simulink model "model_quad_linear_mpc_fail"  (R2021b)
settings: Solver=VariableStepAuto  StartTime=0.0  StopTime=10  RelTol=1e-3
values from neighbouring files (symbols this model uses):
  A = reshape([mt1,mt2,mt3,mt4,mt5,mt6,mt7,mt8],12,12)    [Jacob.m]    (also in Lineared_SS_model.m = reshape([-1.097500e-06;0.000000e+00;0.000000e+00;-4.432200e-; find_optimal_lqr.m = reshape([-1.097500e-06;0.000000e+00;0.000000e+00;-4.432200e-; start_drone.m = zeros(12))
  B = reshape([mt9,mt10],12,4)    [Jacob.m]    (also in Lineared_SS_model.m = reshape([0.000000e+00;0.000000e+00;0.000000e+00;0.000000e+00; find_optimal_lqr.m = reshape([0.000000e+00;0.000000e+00;0.000000e+00;0.000000e+00; nlStateFcn.m = [0 0 0]; start_drone.m = zeros(12,4))
libraries: mpclib x1
settings Model: Creator=Elena  LastModifiedBy=Elena

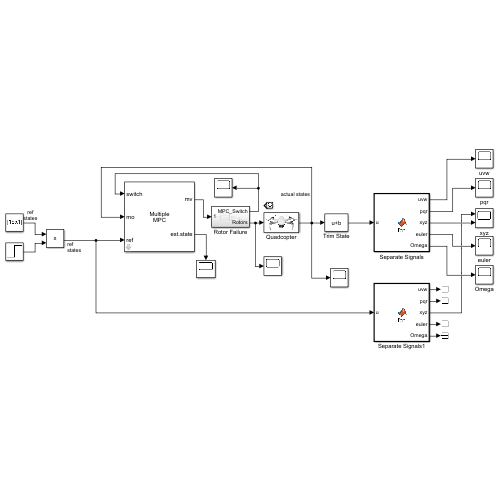
[thumbnail: Simulink's stored preview of the top-level diagram]
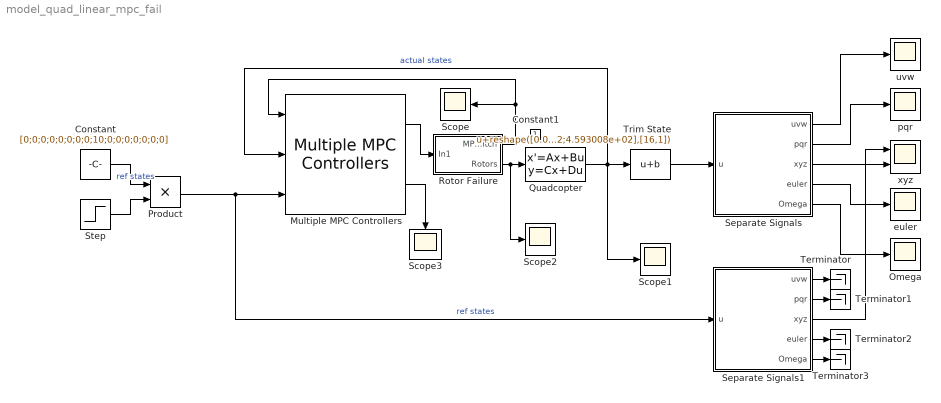
== system model_quad_linear_mpc_fail ==
  Constant : Constant  Value=[0;0;0;0;0;0;0;0;10;0;0;0;0;0;0;0]
  Constant1 : Constant
  Multiple MPC Controllers : mpclib/Multiple MPC Controllers  mpcobjs={'mpc_l','mpc_l_fail_1','mpc_l_fail_2','mpc_l_fail_3','mpc_l_fail_4'}  x0s={'[]','[]','[]','[]','[]'}  Nmpc=1  theMPC=1  nmv=1  nmo=1  nmd=1  nts=1  md_inport_multiple=off  mv_inport_multiple=off  uref_inport_multiple=off  return_cost_multiple=off  return_mvseq_multiple=off  return_qpstatus_multiple=off  return_xseq_multiple=off  return_state_multiple=on  return_ovseq_multiple=off  state_inport_multiple=off  umin_inport_multiple=off  umax_inport_multiple=off  ymin_inport_multiple=off  ymax_inport_multiple=off  ywt_inport_multiple=off  uwt_inport_multiple=off  duwt_inport_multiple=off  rhoeps_inport_multiple=off  BlockDataType_multiple=double  SampleTimeInherited_multiple=off
      settings: SourceProductBaseCode=MP
  Omega : Scope
  Product : Product
  Quadcopter : StateSpace  A=A  B=B  C=eye(16)  D=zeros(16,4)  InitialCondition=0
      mask Display: image('drone_model.png'); % Use "Edit Image" on toolstrip to change.
  Rotor Failure : Subsystem
  Scope{,1..3} (4 alike) : Scope
  Separate Signals : MATLAB Function  TreatAsAtomicUnit=on
  Separate Signals1 : MATLAB Function  TreatAsAtomicUnit=on
  Step : Step  SampleTime=0
  Terminator{,1..3} (4 alike) : Terminator
  Trim State : Bias  Bias=reshape([0.000000e+00;0.000000e+00;0.000000e+00;0.000000e+00;0.000000e+00;0.000000e+00;0.000000e+00;0.000000e+00;0.000000e+00;0.000000e+00;0.000000e+00;0.000000e+00;0;4.593008e+02;4.593008e+02;4.593008e+02],[16,1])
  euler : Scope
  pqr : Scope
  uvw : Scope
  xyz : Scope  NumInputPorts=2
  wires:
  Step/1 -> Product/2
  Quadcopter/1 -> Multiple MPC Controllers/2, Trim State/1, Scope1/1  "actual states"
  Separate Signals/3(xyz) -> xyz/2
  Separate Signals/2(pqr) -> pqr/1
  Separate Signals/1(uvw) -> uvw/1
  Separate Signals/4(euler) -> euler/1
  Separate Signals/5(Omega) -> Omega/1
  Trim State/1 -> Separate Signals/1(u)
  Separate Signals1/3(xyz) -> xyz/1
  Separate Signals1/1(uvw) -> Terminator/1
  Separate Signals1/2(pqr) -> Terminator1/1
  Separate Signals1/4(euler) -> Terminator2/1
  Separate Signals1/5(Omega) -> Terminator3/1
  Multiple MPC Controllers/1 -> Rotor Failure/1(In1)
  Product/1 -> Multiple MPC Controllers/3, Separate Signals1/1(u)  "ref states"
  Constant/1 -> Product/1  "ref states"
  Rotor Failure/2(Rotors) -> Scope2/1, Quadcopter/1
  Rotor Failure/1(MPC_Switch) -> Scope/1, Multiple MPC Controllers/1
  Multiple MPC Controllers/2 -> Scope3/1

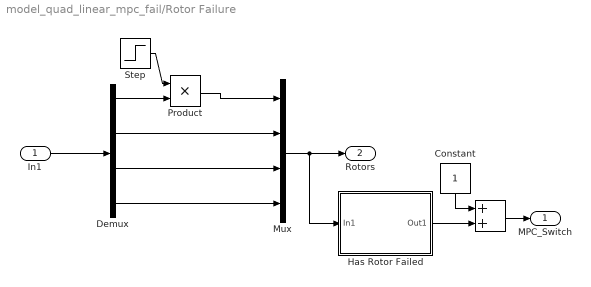
== system model_quad_linear_mpc_fail/Rotor Failure ==
  In1 : Inport
  " " : Sum
  Constant : Constant
  Demux : Demux
  Has Rotor Failed : Subsystem
  Mux : Mux
  Product : Product
  Step : Step  Time=6  Before=1  After=0  SampleTime=0
  MPC_Switch : Outport
  Rotors : Outport  Port=2
  wires:
  In1/1 -> Demux/1
  Demux/3 -> Mux/3
  Demux/4 -> Mux/4
  Product/1 -> Mux/1
  Step/1 -> Product/1
  Demux/2 -> Mux/2
  Demux/1 -> Product/2
  " "/1 -> MPC_Switch/1
  Constant/1 -> " "/1
  Mux/1 -> Has Rotor Failed/1(In1), Rotors/1
  Has Rotor Failed/1(Out1) -> " "/2

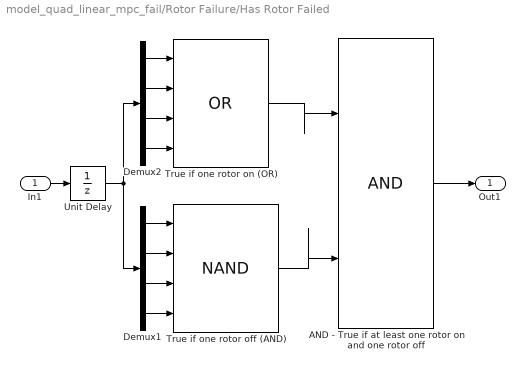
== system model_quad_linear_mpc_fail/Rotor Failure/Has Rotor Failed ==
  In1 : Inport
  "AND - True if at least one rotor on and one rotor off " : Logic  IconShape=distinctive  AllPortsSameDT=off  OutDataTypeStr=boolean
  Demux1 : Demux
  Demux2 : Demux
  True if one rotor off (AND) : Logic  Operator=NAND  Inputs=4  IconShape=distinctive  AllPortsSameDT=off  OutDataTypeStr=boolean
  True if one rotor on (OR) : Logic  Operator=OR  Inputs=4  IconShape=distinctive  AllPortsSameDT=off  OutDataTypeStr=boolean
  Unit Delay : UnitDelay  SampleTime=-1  HasFrameUpgradeWarning=on
  Out1 : Outport
  wires:
  Demux1/2 -> True if one rotor off (AND)/2
  Demux1/4 -> True if one rotor off (AND)/4
  Demux1/1 -> True if one rotor off (AND)/1
  Demux1/3 -> True if one rotor off (AND)/3
  True if one rotor off (AND)/1 -> "AND - True if at least one rotor on and one rotor off "/2
  "AND - True if at least one rotor on and one rotor off "/1 -> Out1/1
  True if one rotor on (OR)/1 -> "AND - True if at least one rotor on and one rotor off "/1
  Unit Delay/1 -> Demux1/1, Demux2/1
  Demux2/3 -> True if one rotor on (OR)/3
  Demux2/1 -> True if one rotor on (OR)/1
  Demux2/4 -> True if one rotor on (OR)/4
  Demux2/2 -> True if one rotor on (OR)/2
  In1/1 -> Unit Delay/1

== matlab function model_quad_linear_mpc_fail/Separate Signals1 ==
  data: u input; uvw output; pqr output; xyz output; euler output; Omega output
function [uvw,pqr,xyz,euler,Omega] = fcn(u)

uvw=u(1:3);
pqr=u((1:3)+3);
xyz=u((1:3)+6);
euler=u((1:3)+9);
Omega=u((1:4)+12);

== matlab function model_quad_linear_mpc_fail/Separate Signals ==
  data: u input; uvw output; pqr output; xyz output; euler output; Omega output
function [uvw,pqr,xyz,euler,Omega] = fcn(u)

uvw=u(1:3);
pqr=u((1:3)+3);
xyz=u((1:3)+6);
euler=u((1:3)+9);
Omega=u((1:4)+12);
